simulink model "trim_sys"  (R2016a)
settings: Solver=VariableStepAuto  StartTime=0.0  StopTime=10.0  RelTol=1e-3
settings Model: Creator=andreanv  LastModifiedBy=andreanv

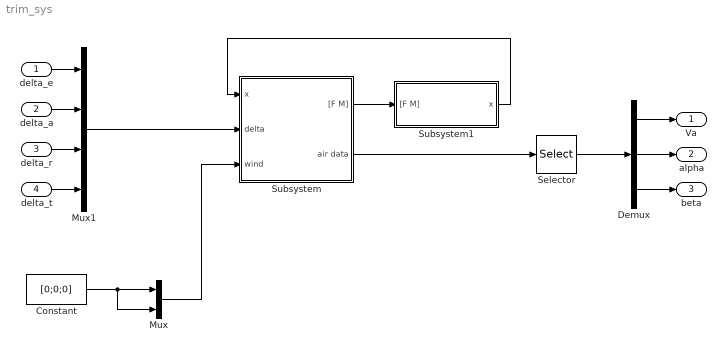
== system trim_sys ==
  delta_e : Inport
  delta_a : Inport  Port=2
  delta_r : Inport  Port=3
  delta_t : Inport  Port=4
  Constant : Constant  Value=[0;0;0]
  Demux : Demux  Outputs=3
  Mux : Mux  Inputs=2
  Mux1 : Mux
  Selector : Selector  InputPortWidth=3  IndexOptions=Index vector (dialog)  Indices=[1 3]  OutputSizes=1
  Subsystem : Subsystem
  Subsystem1 : Subsystem
  Va : Outport
  alpha : Outport  Port=2
  beta : Outport  Port=3
  wires:
  delta_t/1 -> Mux1/4
  delta_r/1 -> Mux1/3
  delta_a/1 -> Mux1/2
  delta_e/1 -> Mux1/1
  Selector/1 -> Demux/1
  Subsystem/2(air data) -> Selector/1
  Demux/3 -> beta/1
  Demux/2 -> alpha/1
  Demux/1 -> Va/1
  Mux/1 -> Subsystem/3(wind)
  Mux1/1 -> Subsystem/2(delta)
  Constant/1 -> Mux/2, Mux/1
  Subsystem/1("[F M]") -> Subsystem1/1("[F M]")
  Subsystem1/1(x) -> Subsystem/1(x)

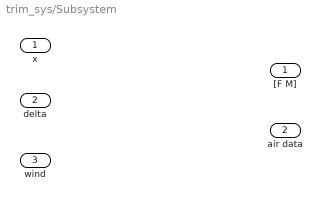
== system trim_sys/Subsystem ==
  x : Inport
  delta : Inport  Port=2
  wind : Inport  Port=3
  "[F M]" : Outport
  air data : Outport  Port=2

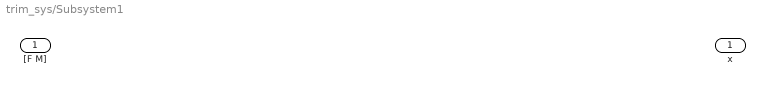
== system trim_sys/Subsystem1 ==
  "[F M]" : Inport
  x : Outport
